simulink model "Ques7Ex1_AkankshaMurali"  (R2023b)
settings: Solver=VariableStepAuto  StartTime=0.0  StopTime=10.0  RelTol=1e-3
settings Model: Creator=akank  LastModifiedBy=akank

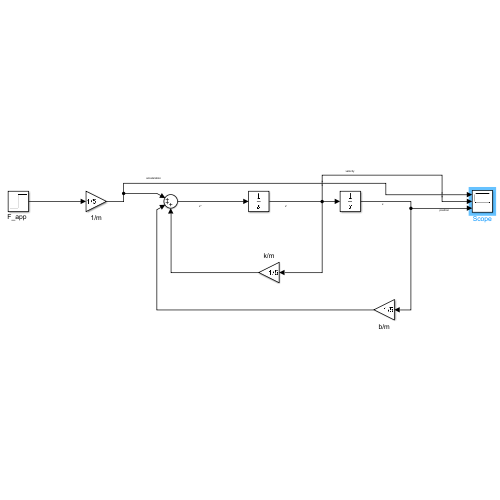
[thumbnail: Simulink's stored preview of the top-level diagram]
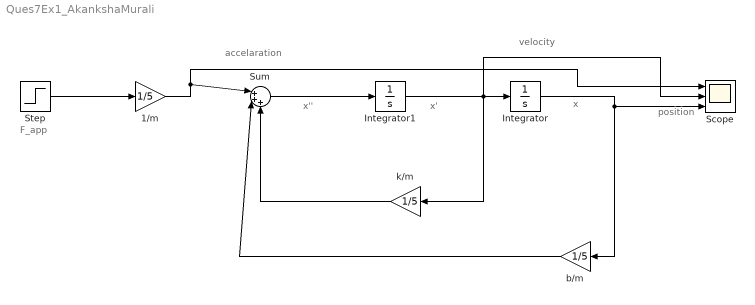
== system Ques7Ex1_AkankshaMurali ==
  note: F_app
  note: accelaration
  note: velocity
  note: position
  note: x''
  note: x'
  note: x
  1/m : Gain  Gain=1/5
  Integrator : Integrator
  Integrator1 : Integrator
  Scope : Scope  NumInputPorts=3
  Step : Step  After=20  SampleTime=0
  Sum : Sum  Inputs=|+++
  b/m : Gain  Gain=1/5
  k/m : Gain  Gain=1/5
  wires:
  Step/1 -> 1/m/1
  1/m/1 -> Scope/1, Sum/1
  Sum/1 -> Integrator1/1
  Integrator1/1 -> Integrator/1, Scope/2, k/m/1
  Integrator/1 -> Scope/3, b/m/1
  k/m/1 -> Sum/3
  b/m/1 -> Sum/2
